simulink model "Exemplu_figura3"  (R2016a)
settings: Solver=VariableStepDiscrete  StartTime=0.0  StopTime=10.0  RelTol=1e-3
undefined symbols (not defined in the file): m
settings Model: Creator=Cristina  LastModifiedBy=Cristina

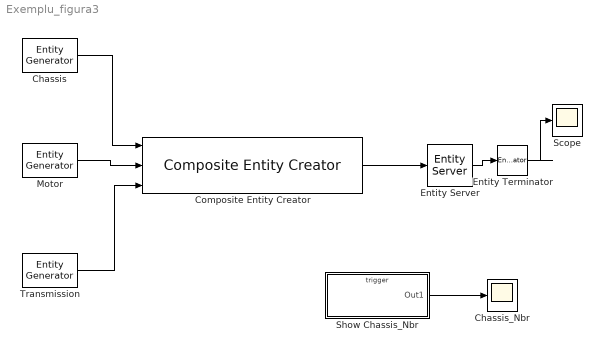
== system Exemplu_figura3 ==
  Chassis : EntityGenerator  OutputPortMessageModes=m  AttributeName=Chassis_Nbr  EntityType=Structured  EntityTypeName=Chassis
  Chassis_Nbr : Scope
  Composite Entity Creator : CompositeEntityCreator  InputPortMessageModes=m,m,m  OutputPortMessageModes=m  NumberInputPorts=3  EntityTypeName=Combined  InputEntityName=Chassis|Motor|Transmission
      settings: InputPortMap=u0,u1,u2
  Entity Server : EntityServer  InputPortMessageModes=m  OutputPortMessageModes=m  Capacity=1  EntryAction=|
      | entity.Chassis.Chassis_Nbr = entity.Motor.Motor_Nbr + 10 * entity.Transmission.Transmission_Nbr;
      | f(entity.Chassis.Chassis_Nbr);
  Entity Terminator : EntityTerminator  InputPortMessageModes=m  NumberEntitiesArrived=on
      settings: OutputPortMap=o0
  Motor : EntityGenerator  OutputPortMessageModes=m  Period=0.3  GenerateAction=|  AttributeName=Motor_Nbr  EntityType=Structured  EntityTypeName=Motor
      | persistent Motor_count
      | if (isempty(Motor_count))
      |     Motor_count = 0;
      | end
      | Motor_count = Motor_count + 1;
      | entity.Motor_Nbr = Motor_count;
  Scope : Scope
  Show Chassis_Nbr : Subsystem  TreatAsAtomicUnit=on
  Transmission : EntityGenerator  OutputPortMessageModes=m  Period=0.5  GenerateAction=|  AttributeName=Transmission_Nbr  EntityType=Structured  EntityTypeName=Transmission
      | persistent Transmission_count
      | if (isempty(Transmission_count))
      |     Transmission_count = 0;
      | end
      | Transmission_count = Transmission_count + 1;
      | entity.Transmission_Nbr = Transmission_count;
  wires:
  Chassis/1 -> Composite Entity Creator/1
  Motor/1 -> Composite Entity Creator/2
  Transmission/1 -> Composite Entity Creator/3
  Composite Entity Creator/1 -> Entity Server/1
  Entity Server/1 -> Entity Terminator/1
  Entity Terminator/1 -> Scope/1
  Show Chassis_Nbr/1(Out1) -> Chassis_Nbr/1

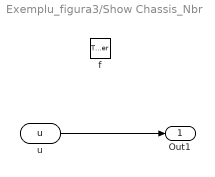
== system Exemplu_figura3/Show Chassis_Nbr ==
  f : TriggerPort  TriggerType=function-call  IsSimulinkFunction=on  FunctionName=f  VariantControl=Variant
  u : ArgIn  DisableCoverage=on  ArgumentName=u
  Out1 : Outport
  wires:
  u/1 -> Out1/1
